simulink model "PID_Motor"  (R2018a)
settings: Solver=VariableStepAuto  StartTime=0.0  StopTime=10  MaxStep=0.01  RelTol=0.001
undefined symbols (not defined in the file or in its folder): k
settings Model: Creator=lucae  LastModifiedBy=lucaerviati
settings SolverCC: MaxConsecutiveMinStep=2

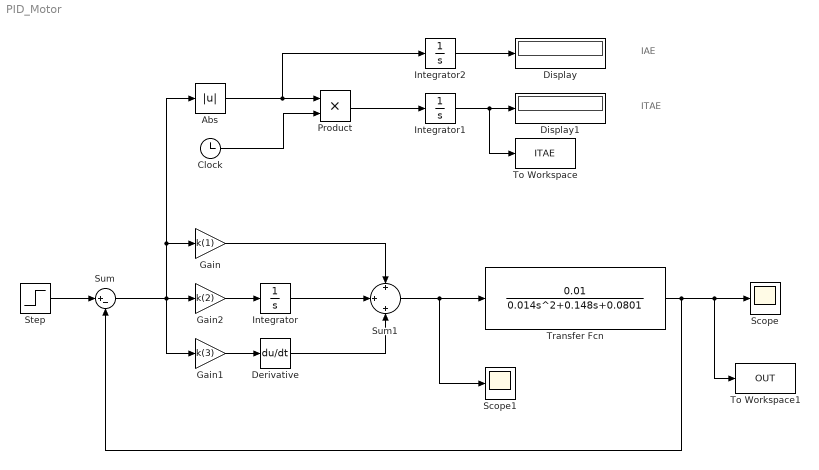
== system PID_Motor ==
  note: IAE
  note: ITAE
  Abs : Abs
  Clock : Clock
  Derivative : Derivative
  Display : Display
  Display1 : Display
  Gain : Gain  Gain=k(1)
  Gain1 : Gain  Gain=k(3)
  Gain2 : Gain  Gain=k(2)
  Integrator : Integrator
  Integrator1 : Integrator
  Integrator2 : Integrator
  Product : Product
  Scope : Scope
  Scope1 : Scope
  Step : Step  SampleTime=0
  Sum : Sum  Inputs=|+-
  Sum1 : Sum  Inputs=+|+|+
  To Workspace : ToWorkspace  VariableName=ITAE  SampleTime=-1
  To Workspace1 : ToWorkspace  VariableName=OUT  SaveFormat=Timeseries  SampleTime=-1
  Transfer Fcn : TransferFcn  Numerator=[0.01]  Denominator=[0.014 0.148 0.0801]
  wires:
  Gain2/1 -> Integrator/1
  Gain1/1 -> Derivative/1
  Sum/1 -> Gain1/1, Gain2/1, Abs/1, Gain/1
  Derivative/1 -> Sum1/3
  Integrator/1 -> Sum1/2
  Gain/1 -> Sum1/1
  Sum1/1 -> Scope1/1, Transfer Fcn/1
  Step/1 -> Sum/1
  Abs/1 -> Integrator2/1, Product/1
  Clock/1 -> Product/2
  Product/1 -> Integrator1/1
  Integrator1/1 -> To Workspace/1, Display1/1
  Integrator2/1 -> Display/1
  Transfer Fcn/1 -> To Workspace1/1, Scope/1, Sum/2
